simulink model "qep_calibration_algorithm"  (R2025b)
settings: Solver=FixedStepDiscrete  StartTime=0.0  StopTime=10.0  RelTol=1e-3
InitFcn:
  | qep_calibration_data;
values from neighbouring files (symbols this model uses):
  PWM_frequency = 20e3    (= 20000)    [qep_calibration_data.m]
  Ts = T_pwm    (= 5e-05)    [qep_calibration_data.m]
undefined symbols (not defined in the file or in its folder): motor
libraries: mcbcontrolslib x3, simulink x2, mcbpositiondecoderlib x2, mcbeeMathTransformLib x1

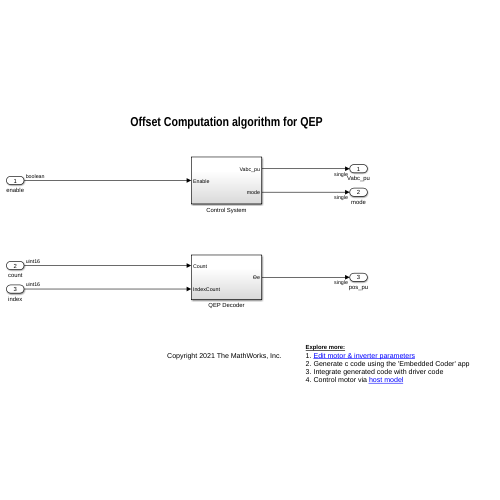
[thumbnail: Simulink's stored preview of the top-level diagram]
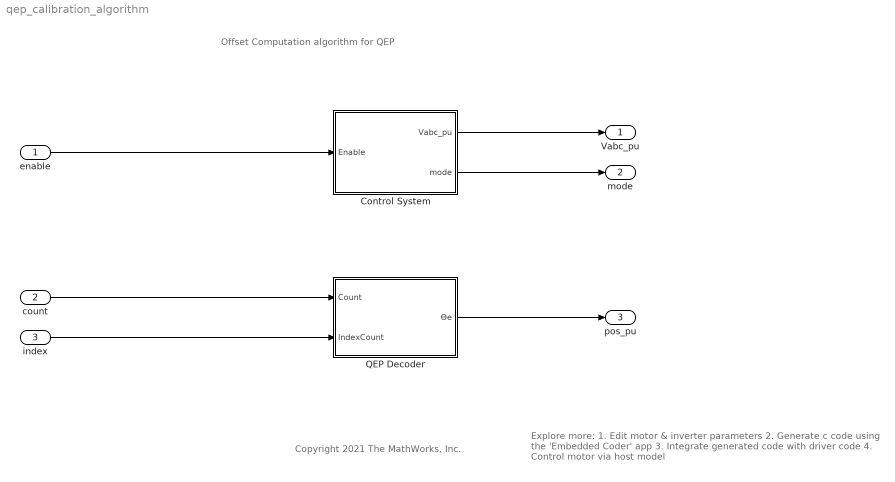
== system qep_calibration_algorithm ==
  note: Offset Computation algorithm for QEP
  note: Explore more:
      | 1. Edit motor & inverter parameters
      | 2. Generate c code using the 'Embedded Coder' app
      | 3. Integrate generated code with driver code
      | 4. Control motor via host model
  note: Copyright 2021 The MathWorks, Inc.
  enable : Inport  OutDataTypeStr=boolean
  count : Inport  Port=2  OutDataTypeStr=uint16
  index : Inport  Port=3  OutDataTypeStr=uint16
  Control System : Subsystem
  QEP Decoder : Subsystem
  Vabc_pu : Outport  OutDataTypeStr=dataType  VectorParamsAs1DForOutWhenUnconnected=off
  mode : Outport  Port=2  OutDataTypeStr=dataType
  pos_pu : Outport  Port=3  OutDataTypeStr=dataType
  wires:
  enable/1 -> Control System/1(Enable)
  Control System/1(Vabc_pu) -> Vabc_pu/1
  Control System/2(mode) -> mode/1
  count/1 -> QEP Decoder/1(Count)
  index/1 -> QEP Decoder/2(IndexCount)
  QEP Decoder/1(ϴe) -> pos_pu/1

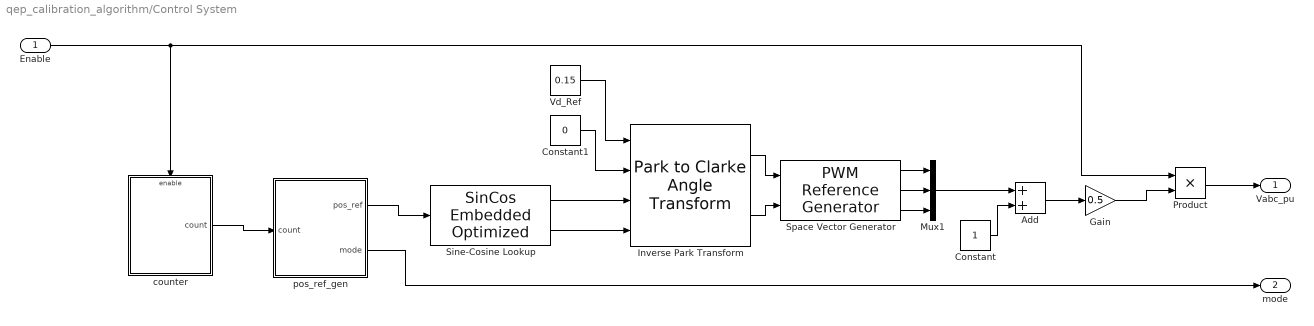
== system qep_calibration_algorithm/Control System ==
  Enable : Inport
  Add : Sum
  Constant : Constant  OutDataTypeStr=dataType
  Constant1 : Constant  Value=0  OutDataTypeStr=dataType  SampleTime=-1
  Gain : Gain  Gain=0.5  OutDataTypeStr=Inherit: Same as input
  Inverse Park Transform : mcbeeMathTransformLib/Park to Clarke Angle Transform  AxisAlignment=D-axis  UseWithEmbedded=on  PhaseInput=Two inputs  ThetaInput=Sine and Cosine electrical position  AngleInput=Per-unit  N_points=1024
  Mux1 : Mux  Inputs=3
  Product : Product  OutDataTypeStr=dataType
  Sine-Cosine Lookup : mcbcontrolslib/SinCos Embedded Optimized  LabelModeActiveChoice=MCB_Sin  OptforProc=off  ApproximationMethod=None  UserApproxMethod=Lookup  ApproxStatus=None  InterpMethod=Linear point-slope  NumberOfDataPoints=16  NumberOfIterations=11  RemoveProtectionAgainstOutOfRangeInput=off  TableDataTypeStr=Inherit: Inherit via input  AngleInput=Per-unit  ThetaDataType=single  N_points=1024  DatatypeInput=Inherit from input  Datatype=Inherit: Same as input
  Space Vector Generator : mcbcontrolslib/PWM Reference Generator  inSignal=Valphabeta  modType=SVM: space vector modulation
  Vd_Ref : Constant  Value=0.15  OutDataTypeStr=dataType  SampleTime=-1
  counter : Subsystem
  pos_ref_gen : Subsystem
  Vabc_pu : Outport
  mode : Outport  Port=2
  wires:
  Sine-Cosine Lookup/2 -> Inverse Park Transform/4
  Inverse Park Transform/2 -> Space Vector Generator/2
  counter/1(count) -> pos_ref_gen/1(count)
  Space Vector Generator/3 -> Mux1/3
  Enable/1 -> counter/Enable, Product/1
  Vd_Ref/1 -> Inverse Park Transform/1
  Constant1/1 -> Inverse Park Transform/2
  Product/1 -> Vabc_pu/1
  Mux1/1 -> Add/1
  pos_ref_gen/1(pos_ref) -> Sine-Cosine Lookup/1
  Sine-Cosine Lookup/1 -> Inverse Park Transform/3
  Space Vector Generator/2 -> Mux1/2
  Inverse Park Transform/1 -> Space Vector Generator/1
  Gain/1 -> Product/2
  Space Vector Generator/1 -> Mux1/1
  pos_ref_gen/2(mode) -> mode/1
  Constant/1 -> Add/2
  Add/1 -> Gain/1

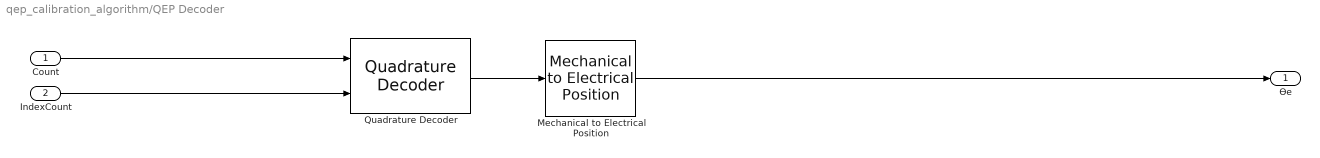
== system qep_calibration_algorithm/QEP Decoder ==
  Count : Inport
  IndexCount : Inport  Port=2
  Mechanical to Electrical Position : mcbpositiondecoderlib/Mechanical to Electrical Position  PolePairsInputType=Specify via dialog  NrPP=motor.polepairs  selectedRange=Per unit  MechOfstInputType=Specify via dialog  mechOffsetIn=0  maxAngleIn=1  InputDataType=dataType  VariantSelect=floating-point
  Quadrature Decoder : mcbpositiondecoderlib/Quadrature Decoder  ParameterInputType=off  CountsPerRevInverseDataType=single  EncoderSlitsPerRevolution=motor.QEPSlits  EncoderCountsPerSlit=4  CounterSize=16 bits  ExternalIndexCount=on  PositionUnit=Per unit  PositionDataType=dataType
  ϴe : Outport
  wires:
  IndexCount/1 -> Quadrature Decoder/2
  Mechanical to Electrical Position/1 -> ϴe/1
  Quadrature Decoder/1 -> Mechanical to Electrical Position/1
  Count/1 -> Quadrature Decoder/1

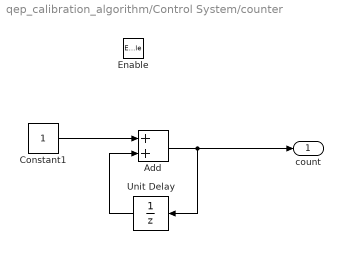
== system qep_calibration_algorithm/Control System/counter ==
  Enable : EnablePort  StatesWhenEnabling=reset
  Add : Sum
  Constant1 : Constant  OutDataTypeStr=uint32
  Unit Delay : UnitDelay  SampleTime=-1  HasFrameUpgradeWarning=on
  count : Outport  InitialOutput=0
  wires:
  Unit Delay/1 -> Add/2
  Constant1/1 -> Add/1
  Add/1 -> count/1, Unit Delay/1

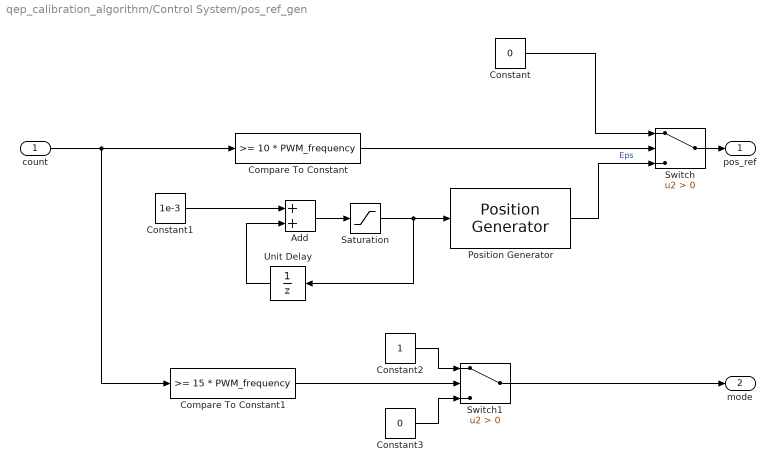
== system qep_calibration_algorithm/Control System/pos_ref_gen ==
  count : Inport
  Add : Sum  OutDataTypeStr=single
  Compare To Constant : simulink/Logic and Bit Operations/Compare To Constant  relop=>=  const=10 * PWM_frequency  OutDataTypeStr=boolean
  Compare To Constant1 : simulink/Logic and Bit Operations/Compare To Constant  relop=>=  const=15 * PWM_frequency  OutDataTypeStr=boolean
  Constant : Constant  Value=0  OutDataTypeStr=dataType
  Constant1 : Constant  Value=1e-3  OutDataTypeStr=dataType
  Constant2 : Constant  OutDataTypeStr=dataType
  Constant3 : Constant  Value=0  OutDataTypeStr=dataType
  Position Generator : mcbcontrolslib/Position Generator  AngleOutput=Per-unit  InitialThetaSource=Specify via dialog  ExternalReset=none  Offset=0
  Saturation : Saturate  UpperLimit=motor.polepairs * Ts
  Switch : Switch  Criteria=u2 > Threshold  SaturateOnIntegerOverflow=off  InputSameDT=off
  Switch1 : Switch  Criteria=u2 > Threshold  SaturateOnIntegerOverflow=off  InputSameDT=off
  Unit Delay : UnitDelay  SampleTime=-1  HasFrameUpgradeWarning=on
  pos_ref : Outport
  mode : Outport  Port=2
  wires:
  Position Generator/1 -> Switch/3  "Eps"
  Constant/1 -> Switch/1
  Switch/1 -> pos_ref/1
  Add/1 -> Saturation/1
  Compare To Constant/1 -> Switch/2
  Unit Delay/1 -> Add/2
  Constant1/1 -> Add/1
  count/1 -> Compare To Constant1/1, Compare To Constant/1
  Compare To Constant1/1 -> Switch1/2
  Constant2/1 -> Switch1/1
  Constant3/1 -> Switch1/3
  Switch1/1 -> mode/1
  Saturation/1 -> Position Generator/1, Unit Delay/1
